simulink model "eulerSIM"  (R2015a)
settings: Solver=ode113  StartTime=0.0  StopTime=t_total  RelTol=1e-3
values from neighbouring files (symbols this model uses):
  A0 = zeros(3,3)    [PS2.m]    (also in PS3.m = getDCM(triad1, triad2); PS4.m = getDCM(triad1, triad2); PS5.m = getDCM(triad1, triad2); PS7.m = getDCM(triad1, triad2))
  I_principle = S_top.tauCM_P    [PS2.m]    (also in PS3.m; PS4.m; PS5.m; PS7.m)
  M0 = [0 0 0]'    [PS2.m]    (also in PS3.m; PS4.m; PS5.m; PS7.m)
  q0 = DCM2Quat_3rdTry(A0)    [PS3.m]
  w0 = w0_28    [PS2.m]    (also in PS3.m = [0; 0; 10/180*pi*rand()]; PS4.m = w0 + 0.0007*[1 1 1]'; PS5.m = [0 -n0 0]'; PS7.m = [0 -2 0]')
settings Model: Creator=Toby  LastModifiedBy=Toby
settings DataIOCC: SaveTime=off

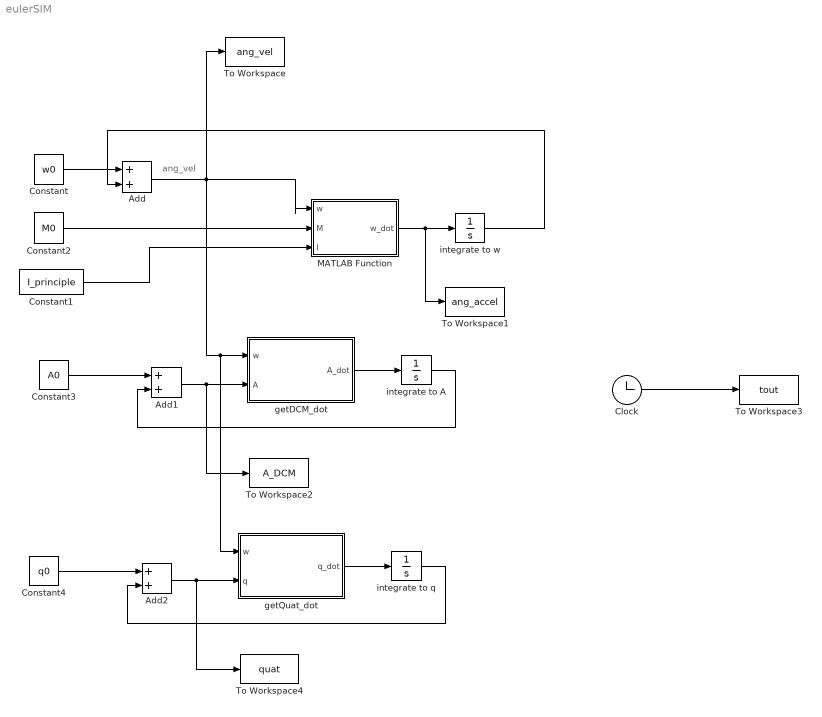
== system eulerSIM ==
  note: ang_vel
  Add : Sum
  Add1 : Sum
  Add2 : Sum
  Clock : Clock
  Constant : Constant  Value=w0
  Constant1 : Constant  Value=I_principle
  Constant2 : Constant  Value=M0
  Constant3 : Constant  Value=A0
  Constant4 : Constant  Value=q0
  MATLAB Function : MATLAB Function  TreatAsAtomicUnit=on
  To Workspace : ToWorkspace  VariableName=ang_vel  SampleTime=-1
  To Workspace1 : ToWorkspace  VariableName=ang_accel  SampleTime=-1
  To Workspace2 : ToWorkspace  VariableName=A_DCM  SampleTime=-1
  To Workspace3 : ToWorkspace  VariableName=tout  SampleTime=-1
  To Workspace4 : ToWorkspace  VariableName=quat  SampleTime=-1
  getDCM_dot : MATLAB Function  TreatAsAtomicUnit=on
  getQuat_dot : MATLAB Function  TreatAsAtomicUnit=on
  integrate to A : Integrator
  integrate to q : Integrator
  integrate to w : Integrator
  wires:
  Constant/1 -> Add/1
  Add/1 -> getQuat_dot/1(w), getDCM_dot/1(w), To Workspace/1, MATLAB Function/1(w)
  integrate to w/1 -> Add/2
  Constant1/1 -> MATLAB Function/3(I)
  Constant2/1 -> MATLAB Function/2(M)
  MATLAB Function/1(w_dot) -> To Workspace1/1, integrate to w/1
  getDCM_dot/1(A_dot) -> integrate to A/1
  integrate to A/1 -> Add1/2
  Add1/1 -> To Workspace2/1, getDCM_dot/2(A)
  Constant3/1 -> Add1/1
  Clock/1 -> To Workspace3/1
  getQuat_dot/1(q_dot) -> integrate to q/1
  integrate to q/1 -> Add2/2
  Add2/1 -> To Workspace4/1, getQuat_dot/2(q)
  Constant4/1 -> Add2/1

== matlab function eulerSIM/getDCM_dot ==
  data: w input; A_dot output; A input
function A_dot   = getDCM_dot( w, A )
%GETDCM_DOT calculate time-derivative of DCM
% w is ang vel of body axes w.r.t. inertial
A_dot = -[0 -w(3) w(2); w(3) 0 -w(1); -w(2) w(1) 0]*A;

end

== matlab function eulerSIM/MATLAB Function ==
  data: w input; w_dot output; M input; I input
function w_dot = eulerRHS(w, M, I)
% principle axis euler eq
% w is 3x1 rotational velocity
% M is 3x1 external torques
Ix = I(1,1); Iy = I(2,2); Iz = I(3,3);
w_dot = zeros(3,1);
w_dot(1) = (M(1) - (Iz - Iy)*w(2)*w(3) ) / Ix;
w_dot(2) = (M(2) - (Ix - Iz)*w(1)*w(3) ) / Iy;
w_dot(3) = (M(3) - (Iy - Ix)*w(1)*w(2) ) / Iz;
end

== matlab function eulerSIM/getQuat_dot ==
  data: w input; q_dot output; q input
function q_dot   = getQuat_dot( w, q )
%GETDCM_DOT calculate time-derivative of DCM
% w is ang vel of body axes w.r.t. inertial
B = [0 w(3) -w(2) w(1); -w(3) 0 w(1) w(2); w(2) -w(1) 0 w(3); ...
  -w(1) -w(2) -w(3) 0];
q_dot = 0.5 * B * q;
end
